simulink model "deadbeat_smm_with_lqr"  (R2015a)
settings: Solver=FixedStepDiscrete  SolverMode=SingleTasking  StartTime=0.0  StopTime=inf  FixedStep=sample_time  RelTol=1e-3
undefined symbols (not defined in the file or in its folder): A_kalman_fourbar_gear, A_kalman_transverse, A_kalman_vertical, A_lpf_accelerometer, A_lpf_fourbar_angles, A_lpf_imu, A_lpf_lateral_angle, B1_lpf_accelerometer, B1_lpf_fourbar_angles, B1_lpf_imu, B1_lpf_lateral_angle, B2_lpf_accelerometer, B2_lpf_fourbar_angles, B2_lpf_imu, B2_lpf_lateral_angle, B_dx_versus_x0, B_kalman_fourbar_gear, B_kalman_transverse, B_kalman_vertical, backwards_K_sag_of_t, backwards_P_sag_of_t, C_kalman_fourbar_gear, C_kalman_transverse, C_kalman_vertical, com_leg_motor, com_torso, contact_threshold, control_start_time, d_ankle_to_foot, d_vertical_com, desired_com_forward_velocity, desired_com_lateral_velocity, desired_initial_leg_roll_left, desired_initial_leg_roll_right, desired_stance_beta2, desired_standing_torso_pitch, desired_standing_torso_roll, desired_standing_z, desired_torso_pitch, desired_torso_roll, Discrete, enable_bouncing, fcut_contact, fdesignblkfcn, forward_dx_of_dxstar, forward_x_of_dxstar, g, gcbh, HIP_MTR_MAX_CONT_TORQUE, HIP_MTR_MAX_TORQUE, i_leg_motor, i_robot, i_torso, initial_dx_estimate, initial_dy_estimate, initial_dz_estimate, initial_leg_selection, initial_z_estimate, k_lateral_accel_for_torso_roll, k_lateral_swing_on_boom ... (+77)
libraries: simulink x21, ctrlSharedLib x7, dsparch4 x3
(part 5 of 5)

== matlab function deadbeat_smm_with_lqr/Control/Behavior Control/Primary and Lateral Behavior/Flight/Generate Parabolic Foot Trajectories ==
  data: time_remaining input; est_duration input; x_star input; y_star input; x0 input; dx0 input; y0 input; dy0 input; zdz0 input; max_parabolic_z_retraction parameter; flight input; right_left input; z_land parameter; min_f_duration parameter; X_star output size=3; Y_star output size=3; Z_star output size=3; robot_is_attached_to_boom parameter; lateral_target_position_left parameter; lateral_target_position_right parameter
%% Parabolic trajectory generation for x, y, and z
% est_duration: estimated flight time
% time_remaining: time until estimated touchdown
% stance: 1 if in stance, 0 otherwise
% x_star: desired x for foot to COM
% y_star: desired y for foot to COM
% x0: x position at takeoff
% y0: y position at takeoff
% zdz0: [z, dz] at takeoff
% max_retract: how high to lift z for ground clearance
% z_land: nominal z height for landing
% min_f_duration: minimum trajectory time

function [X_star, Y_star, Z_star]  =  ...
          GenerateParabolicFootTrajectory(time_remaining, est_duration,  ...
                               x_star, y_star, x0, dx0, y0, dy0, zdz0, ...
                               max_parabolic_z_retraction,  flight, right_left, ...
                               z_land, min_f_duration, ...
                               robot_is_attached_to_boom, lateral_target_position_left, lateral_target_position_right)

if ~flight
    X_star = [0;0;0];
    Y_star = [0;0;0];
    Z_star = [0;0;0];
    return;
end

if robot_is_attached_to_boom
    if right_left
        y_star = lateral_target_position_right;
    else
        y_star = lateral_target_position_left;
    end 
end
                           
% we are solving for yawed coordinates xyz of com-foot in flight and
% converting them to joint angles

% estimate z ballistically
% z = z_dz_liftoff(1) + z_dz_liftoff(2)*t_flight -g/2*t_flight^2;
% dz = z_dz_liftoff(2) - g*t_flight;
% 
% z = com_xdx_ydy_zdz(5); dz = com_xdx_ydy_zdz(6);
% time_remaining = (-dz-sqrt(max(dz^2 - 4*g/2*(z_land-z), 0) ) )/ (-g); % ballistic estimate of landing


  % plan a traj from init to desired in estimated duration. Use a
  % discontinuous initial condition if estimated duration too short.
  duration = max(est_duration, min_f_duration);
  t_r = max(min(time_remaining, duration),0);
  % sweep a parabola from x0 to x_star with dx_end = -dx0
  dx_star = dx0;
  x_star_t = x_star + dx_star*t_r + (x0-x_star-dx_star*duration)*(t_r/duration)^2;
  dx_star_t = -dx_star - 2*(x0-x_star-dx_star*duration)*(t_r/duration^2);
  ddx_star_t =  2*(x0-x_star-dx_star*duration)*(1/duration^2);
  
  % same for y
  dy_star = dy0;
  y_star_t = y_star + dy_star*t_r + (y0-y_star-dy_star*duration)*(t_r/duration)^2;
  dy_star_t = -dy_star - 2*(y0-y_star-dy_star*duration)*(t_r/duration^2);
  ddy_star_t =  2*(y0-y_star-dy_star*duration)*(1/duration^2);
  
  % Zero out velocities when out of time
  if time_remaining < 0
    dx_star_t = 0; ddx_star_t = 0;
    dy_star_t = 0; ddy_star_t = 0;
  end 
  
  % split duration into thirds.  First segment: parabola from z0 to
  % max_retract.  Second and third segments, cos to landing.
  z0 = zdz0(1);
  dt3 = duration / 3;
  z_min = z_land - max_parabolic_z_retraction;
  if t_r > 2*dt3;
    z_star_t = z_min + (z0-z_min)*((t_r-2*dt3)/dt3)^2;
    dz_star_t = -(z0-z_min)*2*(t_r-2*dt3)/dt3/dt3;
    ddz_star_t = (z0-z_min)*2/dt3^2;
  else
    z_star_t = z_land + (z_min-z_land)/2*(1-cos(t_r/(2*dt3)*pi));
    dz_star_t = -(z_min-z_land)/2*sin(t_r/(2*dt3)*pi)*pi/(2*dt3);
    ddz_star_t = (z_min-z_land)/2*cos(t_r/(2*dt3)*pi)*(pi/(2*dt3))^2;
  end
  
  % track a sinusoidal z of amplitude max_retract, finishing a half-cycle by t_end
  X_star = [x_star_t; dx_star_t; ddx_star_t];
  Y_star = [y_star_t; dy_star_t; ddy_star_t];
  Z_star = [z_star_t; dz_star_t; ddz_star_t];

== matlab function deadbeat_smm_with_lqr/Control/Behavior Control/Primary and Lateral Behavior/Flight/Lateral Flight Control ==
  data: hopping input; tau_primary output; tau_secondary output; RightLeftPrimary input; TorsoRoll input; LLegRoll input; RLegRoll input; Beta1_star input; Roll_star input; K_right_lat_flight parameter; K_left_lat_flight parameter; K_right_lat_flight_winch parameter; K_left_lat_flight_winch parameter; Q_phibeta1beta2 parameter; Q_phibeta1beta2_winch parameter; m_torso parameter; m_leg parameter; m_leg_motor parameter; m_total_real parameter; com_torso parameter; i_torso parameter; i_leg_motor parameter; g parameter; lateral_offset parameter; k_lateral_swing_on_boom parameter; adjusted_ref output; feedforward output; lateral_target_beta parameter; robot_is_attached_to_boom parameter
% full_state = [Roll; Beta1; Beta2; dRoll; dBeta1; dBeta2];
function [tau_primary, tau_secondary, ...
          adjusted_ref, feedforward] = lateral_flight_control(hopping, RightLeftPrimary,...
          TorsoRoll, LLegRoll, RLegRoll, Beta1_star, Roll_star,...
          K_right_lat_flight, K_left_lat_flight, K_right_lat_flight_winch, K_left_lat_flight_winch, Q_phibeta1beta2, Q_phibeta1beta2_winch,...
          m_torso, m_leg, m_leg_motor, m_total_real, com_torso, i_torso, i_leg_motor, g, lateral_offset, ...
          k_lateral_swing_on_boom, lateral_target_beta, robot_is_attached_to_boom)

    %% Define inertial quantities
    d = norm(com_torso(2:3));
    It_f = i_torso(1);
    Im_f = i_leg_motor(1); 
    phidphi = TorsoRoll; 
    symdsym = LLegRoll-RLegRoll;
    ang_mom = phidphi(2)*(m_torso*d^2 + It_f + 2*(m_leg_motor*lateral_offset^2+ Im_f)) -symdsym(2)*(m_leg_motor*lateral_offset^2+Im_f);

    %% Assign desired and measured variables 
    if RightLeftPrimary == 1
        Beta1 = RLegRoll;
        Beta2 = LLegRoll;
        Beta2_star = [lateral_target_beta; 0; 0];
    else
        Beta1 = LLegRoll;
        Beta2 = RLegRoll;
        Beta2_star = [lateral_target_beta; 0; 0];
    end    
    
    %% If robot is still on the winch, use a different set of gains
    if ~hopping
        Q_phibeta1beta2 = Q_phibeta1beta2_winch;
        K_right_lat_flight = K_right_lat_flight_winch;
        K_left_lat_flight = K_left_lat_flight_winch;
    end

    %% LQR
    ref_old = [Roll_star(1); Beta1_star(1); Beta2_star(1)];
    dref_old = [0; Beta1_star(2); Beta2_star(2)];
    ddref_old = [0; Beta1_star(3); Beta2_star(3)];
    
    % eliminate beta2 from state using momentum:
    % s_old = T*s_new+D(t); s_new = [phi; beta1];
    % dbeta_R = L/(Im_f+mm*r^2) - (It_f+mm*d^2+2*Im_f+2*mm*r^2)/(Im_f+mm*r^2)*dphi + dbeta_L 
    % beta_R = beta_R0 + L/(Im_f+mm*r^2)*t - ((It_f+mm*d^2+2*Im_f+2*mm*r^2)/(Im_f+mm*r^2)*(phi-phi0) + (beta_L-beta_L0)
    % beta_R = [beta_R0-b1*phi0-b2*beta_L0 + a*t + b1*phi + b2*beta_L;
    
    if RightLeftPrimary == 1 % beta_2 is beta_L, beta_1 is beta_R, eliminate beta2
      a = -ang_mom/(Im_f+m_leg_motor*lateral_offset^2);
      b1 = (It_f+m_torso*d^2+2*Im_f+2*m_leg_motor*lateral_offset^2)/(Im_f+m_leg_motor*lateral_offset^2); b2 = 1;
    else
      a = +ang_mom/(Im_f+m_leg_motor*lateral_offset^2);
      b1 = -(It_f+m_torso*d^2+2*Im_f+2*m_leg_motor*lateral_offset^2)/(Im_f+m_leg_motor*lateral_offset^2); b2 = 1;
    end
    
    T = [eye(2); b1, b2];
    %  D = [0; 0; 0; 0; beta_R0 - b1*phi0 - b2*beta_L0 + a*t; a];
    D = [0;0; Beta2(1) - b1*phidphi(1) - b2*Beta1(1)];
    
    % old cost (state s)  (s-s_ref)' * Q *(s-s_ref);
    % new cost (state r) =(T*r+D-s_ref)'*Q*(T*r+D-s_ref);
    %                    =(r+ (T'QT)^{-1}T'Q(D-s_ref))'*T'QT*
    %                     (r + (T'QT)^{-1}T'Q(D-s_ref))
    
    
    Q_new = T'*Q_phibeta1beta2*T;
    ref_new = Q_new\T'*Q_phibeta1beta2*(ref_old-D);
    ref_new_vel = Q_new\T'*Q_phibeta1beta2*(dref_old - [0;0; a]);
    ref_accels = Q_new\T'*Q_phibeta1beta2*(ddref_old);

    % A_phidphi_betadbeta1 = [0 1 0 0; 0 0 0 0; 0 0 0 1; 0 0 0 0];
    % assume beta1 is right
    if RightLeftPrimary == 1
        B_new_state = [0 0; 0 0; -1/(It_f+m_torso*d^2), 1/(It_f+m_torso*d^2); 1/(It_f+m_torso*d^2)+1/(Im_f+m_leg_motor*lateral_offset^2), -1/(It_f+m_torso*d^2)];
    else
        B_new_state = [0 0; 0 0; 1/(It_f+m_torso*d^2), -1/(It_f+m_torso*d^2); 1/(It_f+m_torso*d^2)+1/(Im_f+m_leg_motor*lateral_offset^2), -1/(It_f+m_torso*d^2)];
    end      
    
    %   K = lqr(A_phidphi_betadbeta1, B_phidphi_betadbeta1, Q_new, R_lat_flight);
    if RightLeftPrimary == 1
      K = K_right_lat_flight;
    else
      K = K_left_lat_flight;
    end

    new_state = [phidphi(1); Beta1(1); phidphi(2); Beta1(2)];
    new_ref_traj = [ref_new; ref_new_vel];

    feedforward = B_new_state([3 4],:)\ref_accels;
    if ~hopping, feedforward = -(m_leg_motor)*g*lateral_offset*ones(2,1); end
    tau_lqr = feedforward - K*(new_state-new_ref_traj);
    tau_1 = tau_lqr(1); tau_2 = tau_lqr(2);
    implied_beta2_star = [0 0 1]*(T*ref_new+D);
    implied_dbeta2_star = [0 0 1]*(T*ref_new_vel+[0; 0; a]);
    % implied_betadbeta2_star = [0 0 0 0 1 0; 0 0 0 0 0 1]*(T*ref_new+D);
    adjusted_ref = [ref_new; implied_beta2_star; ref_new_vel; implied_dbeta2_star];

    tau_primary = tau_1;
    tau_secondary = tau_2;
    
    
    %% When attached to boom, just do a simple PD control on lateral leg positions
    if robot_is_attached_to_boom
        tau_primary = k_lateral_swing_on_boom'*([lateral_target_beta; 0] - Beta1);
        tau_secondary = k_lateral_swing_on_boom'*([lateral_target_beta; 0] - Beta2);
    end
end

== matlab function deadbeat_smm_with_lqr/Control/Behavior Control/Primary and Lateral Behavior/Flight/Virtual Leg to Four Bar ==
  data: l_leg input; dl_leg input; ddl_leg input; phi input; dphi input; ddphi input; back output; dback output; ddback output; front output; dfront output; ddfront output
function [back, dback, ddback, front, dfront, ddfront] = VirtualLegToFourBar(l_leg, dl_leg, ddl_leg, phi, dphi, ddphi)
    [back, dback, ddback, front, dfront, ddfront] = VirtualLegToFourBar(l_leg, dl_leg, ddl_leg, phi, dphi, ddphi);
end

== matlab function deadbeat_smm_with_lqr/Control/Behavior Control/Primary and Lateral Behavior/Stance/3D Inverse Dynamics yawed ==
  data: right_or_left input; primary_leg_torque output double size=1; primary_leg_force output double size=1; torso_roll input double size=2; torso_pitch input double size=2; torso_yaw input size=2; primary_sagittal_leg_angle input size=2; primary_leg_length input size=2; primary_leg_roll input size=2; secondary_leg_roll input size=2; GRF_desired input double size=3; ddRoll_desired input double size=1; g parameter; primary_lateral_torque output double size=1; secondary_lateral_torque output double size=1; m_leg_motor parameter; m_torso parameter; i_torso parameter; i_leg_motor parameter; lateral_offset parameter; com_torso parameter; torso_centerline_roll_offset_angle parameter
%% Inverse dynamics
function [primary_leg_torque, primary_leg_force, primary_lateral_torque, secondary_lateral_torque]  =  InverseDynamics3D(right_or_left,...
                                                                                                                         torso_roll, torso_pitch, torso_yaw, ...
                                                                                                                         primary_sagittal_leg_angle, primary_leg_length, ...
                                                                                                                         primary_leg_roll, secondary_leg_roll, ...
                                                                                                                         GRF_desired, ddRoll_desired, ...
                                                                                                                         g, m_leg_motor, m_torso, i_torso, i_leg_motor, lateral_offset, com_torso, torso_centerline_roll_offset_angle)

    d = norm(com_torso(2:3));
    It = mean(i_torso);
    Im = mean(i_leg_motor);
    
    phi    = torso_roll(1) + torso_centerline_roll_offset_angle; % roll
    theta  = torso_pitch(1);                   % pitch
    alpha1 = primary_sagittal_leg_angle(1);    % primary sagittal leg angle
    beta1  = primary_leg_roll(1);              % primary leg roll
    beta2  = secondary_leg_roll(1);            % secondary leg roll
    if right_or_left
        beta1 = beta1 - torso_centerline_roll_offset_angle;
        beta2 = beta2 + torso_centerline_roll_offset_angle;
    else
        beta1 = beta1 + torso_centerline_roll_offset_angle;
        beta2 = beta2 - torso_centerline_roll_offset_angle;
    end 
    l1     = primary_leg_length(1);            % primary leg length
    
    dphi    = torso_roll(2);
    dtheta  = torso_pitch(2);
    dpsi    = torso_yaw(2);
    dalpha1 = primary_sagittal_leg_angle(2);
    dbeta1  = primary_leg_roll(2);
    dbeta2  = secondary_leg_roll(2);
    dl1     = primary_leg_length(2);

    Fx = GRF_desired(1);
    Fy = GRF_desired(2);
    Fz = GRF_desired(3);
    ddphi = ddRoll_desired;

    if right_or_left == 1
      A = A_id_roll_yawed_right(lateral_offset,d,m_leg_motor,m_torso,It,Im,phi,theta,alpha1,beta1,beta2,l1);     
      B = B_id_roll_yawed_right(lateral_offset,d,g,m_leg_motor,m_torso,It,Im,phi,theta,alpha1,beta1,beta2,l1,dphi,dtheta,dpsi,dalpha1,dbeta1,dbeta2,dl1,Fx,Fy,Fz,ddphi);
    else
      A = A_id_roll_yawed_left(lateral_offset,d,m_leg_motor,m_torso,It,Im,phi,theta,alpha1,beta1,beta2,l1);     
      B = B_id_roll_yawed_left(lateral_offset,d,g,m_leg_motor,m_torso,It,Im,phi,theta,alpha1,beta1,beta2,l1,dphi,dtheta,dpsi,dalpha1,dbeta1,dbeta2,dl1,Fx,Fy,Fz,ddphi);
    end        
    
    x_id_roll = A \ B;
    primary_leg_torque = x_id_roll(10);
    primary_lateral_torque = x_id_roll(11);
    secondary_lateral_torque = x_id_roll(12);
    primary_leg_force = x_id_roll(13);
end

== matlab function deadbeat_smm_with_lqr/Control/Behavior Control/Primary and Lateral Behavior/Stance/COM X,Y,Z  trajectory generation ==
  data: stance input; hopping input; bouncing input; x_0 output size=1; y_0 output size=1; z_ref output size=1; dz_ref output size=1; ddz_ref output size=1; x_ref output size=1; dx_ref output size=1; y_ref output size=1; dy_ref output size=1; t input size=1; dx0 input; dy0 input; target_DX input; target_DY input; z_rest_new parameter; z_amplitude parameter; spring_frequency parameter; phase_0 parameter; forward_x_of_dxstar parameter; forward_dx_of_dxstar parameter; target_dx_range parameter; T_s parameter; desired_standing_z parameter; standing_bounce_amplitude parameter; standing_bounce_w input; standing_bounce_dw input
%% COM trajectory generation for stance & foot placement for flight

% Outputs:
% x_0: desired x position for COM at touchdown
% y_0: desired y position for COM at touchdown
% [z_ref, dz_ref, ddz_ref]: reference trajectory for vertical
% [x_ref, dx_ref]: reference trajectory for forward
% [y_ref, dy_ref]: reference trajectory for lateral

% Inputs:
% t: time since touchdown
% dx0: touchdown x velocity
% dy0: touchdown y velocity
% target_DX: desired x velocity at takeoff
% s_duration: nominal stance time
% z_rest_new: z height of oscillation
% target_dx_range: full range of possible x velocities in lookup table
% forward_x_of_dxstar: master lookup table for x trajectories
% T_s: tabled vector from 0 to s_duration

function [x_0, y_0,...
          z_ref, dz_ref, ddz_ref, ...
          x_ref, dx_ref, y_ref, dy_ref] ...
          = ReferenceTrajectory(stance, hopping, bouncing, t, dx0, dy0, target_DX, target_DY, z_rest_new, z_amplitude, ...
            spring_frequency, phase_0, forward_x_of_dxstar, forward_dx_of_dxstar, ...
            target_dx_range, T_s,...
            desired_standing_z, standing_bounce_amplitude, standing_bounce_w, standing_bounce_dw)
    
    % Z trajectory 
    z_ref =  z_rest_new + z_amplitude*sin(spring_frequency*t+phase_0);
    dz_ref = z_amplitude*spring_frequency*cos(spring_frequency*t+phase_0);
    ddz_ref = -z_amplitude*spring_frequency^2*sin(spring_frequency*t+phase_0);
    
    % saturate t and initial velocity to reference library
    t_sat = max( min(t, T_s(end)), 0);

    % [X, dX] trajectory from 0 to s_duration
    forward_x_given_dxstar = squeeze(interp1(target_dx_range, forward_x_of_dxstar, target_DX));
    forward_dx_given_dxstar = squeeze(interp1(target_dx_range, forward_dx_of_dxstar, target_DX));

    dx0 = max( min(dx0, max(forward_dx_given_dxstar(:,1))), min(forward_dx_given_dxstar(:,1)) );
    x_ref  = interp2(T_s, forward_dx_given_dxstar(:,1), forward_x_given_dxstar, t_sat, dx0);
    dx_ref = interp2(T_s, forward_dx_given_dxstar(:,1), forward_dx_given_dxstar, t_sat, dx0);
    x_0 = interp1(forward_dx_given_dxstar(:,1), forward_x_given_dxstar(:,1), dx0);

    % [Y, dY] trajectory from 0 to s_duration
    % Y uses same library as X
    forward_y_given_dxstar = squeeze(interp1(target_dx_range, forward_x_of_dxstar, target_DY));
    forward_dy_given_dxstar = squeeze(interp1(target_dx_range, forward_dx_of_dxstar, target_DY));

    dy0 = max( min(dy0, max(forward_dy_given_dxstar(:,1))), min(forward_dy_given_dxstar(:,1)) );
    y_ref  = interp2(T_s, forward_dy_given_dxstar(:,1), forward_y_given_dxstar, t_sat, dy0);
    dy_ref = interp2(T_s, forward_dy_given_dxstar(:,1), forward_dy_given_dxstar, t_sat, dy0);
    y_0 = interp1(forward_dy_given_dxstar(:,1), forward_y_given_dxstar(:,1), dy0);
    
    if ~hopping && ~bouncing % Standing still
        z_ref = desired_standing_z;
        dz_ref = 0;
        ddz_ref = 0;
        x_ref = 0;
        dx_ref = 0;
        y_ref = 0;
        dy_ref =0;
    elseif ~hopping && bouncing % Bouncing while standing
        z_ref = z_rest_new + standing_bounce_amplitude*sin(t*standing_bounce_w);
        dz_ref = standing_bounce_amplitude*cos(t*standing_bounce_w)*(t*standing_bounce_dw + standing_bounce_w);
        ddz_ref = standing_bounce_amplitude*(2*standing_bounce_dw*cos(t*standing_bounce_w) - (t*standing_bounce_dw + standing_bounce_w)^2*sin(t*standing_bounce_w));
        x_ref = 0;
        dx_ref = 0;
        y_ref = 0;
        dy_ref =0;
    end
    if ~stance % Flight
        z_ref = 0;
        dz_ref = 0;
        ddz_ref = 0;
        x_ref = 0;
        dx_ref = 0;
        y_ref = 0;
        dy_ref =0;    
    end
  
end

== matlab function deadbeat_smm_with_lqr/Control/Behavior Control/Primary and Lateral Behavior/Stance/Feedback for Lateral Stabilization ==
  data: Fy_desired output; neutral_feedforward_Fy output; hopping input; stance input; right_left input; rolldroll input; symdsym input; y_dy input; beta2dbeta2 input; z_dz input; GRF_measured input; secondary_lateral_torque_desired output double size=1; m_torso parameter; m_leg_motor parameter; m_leg parameter; lateral_offset parameter; com_torso parameter; i_torso parameter; i_leg_motor parameter; desired_standing_torso_roll parameter; desired_torso_roll parameter; desired_beta2_state input; angular_momentum output; k_stance_secondary_roll parameter; k_lateral_accel_for_torso_roll parameter; g parameter; m_total_real parameter
%  x_front = [y, roll, sym, dy, droll, L]; 
function [Fy_desired,neutral_feedforward_Fy, secondary_lateral_torque_desired, angular_momentum]  =  ...
    FrontalStabilization(hopping, stance, right_left, rolldroll, symdsym, y_dy, beta2dbeta2, z_dz, GRF_measured,...
           m_torso, m_leg_motor, m_leg, lateral_offset, com_torso, i_torso, i_leg_motor, ...
           desired_standing_torso_roll, desired_torso_roll, desired_beta2_state, k_stance_secondary_roll, k_lateral_accel_for_torso_roll, g, m_total_real)
    
    % Angular momentum about the pelvis in the frontal plane
    d = norm(com_torso(2:3));
    It_f = i_torso(1);
    Im_f = i_leg_motor(1);
    lateral_robot_inertia = m_torso*d^2 + It_f + 2*(m_leg_motor*lateral_offset^2+ Im_f);
    angular_momentum = rolldroll(2)*lateral_robot_inertia - symdsym(2)*(m_leg_motor*lateral_offset^2+Im_f);
    
    % Feedforward GRFy for inverse dynamics
    neutral_feedforward_Fy = GRF_measured(3)*y_dy(1)/z_dz(1);
    
    % Desired states
    if hopping
        desired_torso_roll_state = [desired_torso_roll; 0]; 
    else
        desired_torso_roll_state = [desired_standing_torso_roll; 0];
    end
    
    % Motor torque commands
    ddz = GRF_measured(3) / m_total_real - g;
    gravity_comp = (m_leg_motor+m_leg)*lateral_offset*ddz;
    secondary_lateral_torque_desired = k_stance_secondary_roll'*(desired_beta2_state - beta2dbeta2) + gravity_comp;
    feedback_Fy = (lateral_robot_inertia * k_lateral_accel_for_torso_roll*(desired_torso_roll_state - rolldroll)) / z_dz(1);
    Fy_desired =  neutral_feedforward_Fy + feedback_Fy;
    Fy_desired = min(max(Fy_desired, -0.5*abs(GRF_measured(3))), 0.5*abs(GRF_measured(3)));
    
    if ~stance
        Fy_desired = 0;
        secondary_lateral_torque_desired = 0;
        neutral_feedforward_Fy = 0;
    end
end

== matlab function deadbeat_smm_with_lqr/Control/Behavior Control/Primary and Lateral Behavior/Stance/LQR Feedback for Desired Forward GRF ==
  data: hopping input; stance input; GRFx_desired output; netural_pitch_ff output; true_ff output; GRFx_lqr output; ddtheta_star output; ddtheta_star_neutral output; xdx input; thetadtheta input; zdz input; Fz_desired input; xdx_ref input size=2; theta_star input; K_sag input; P_sag input; measured_GRF input; Fx_disturbance input; i_robot parameter; cost_to_go output double size=1; ang_mom output; desired_standing_torso_pitch parameter; k_LQR_sagittal_infinite parameter; P_LQR_sagittal_infinite parameter
%% LQR for x state

% stance: 1 if in stance, 0 otherwise
% xdx: [ x from stance leg to COM, dx of COM]
% thetadtheta: [pitch, dpitch]
% zdz: [z of COM, dz of COM]
% Fz: Desired z GRF
% xdx_ref: [x, dx] current reference point for COM
% theta_star: desired torso pitch
% K_sag: time dependent LQR gain


% sagittal_state: [x, pitch, dx, dptich]
% theta_star: desired torso pitch


function [GRFx_desired, netural_pitch_ff, true_ff, GRFx_lqr, ddtheta_star, ddtheta_star_neutral, cost_to_go, ang_mom]  =  ...
    LQR_Sagittal(hopping, stance, xdx, thetadtheta, zdz, Fz_desired, xdx_ref, theta_star, K_sag, P_sag, measured_GRF, Fx_disturbance, i_robot,...
    desired_standing_torso_pitch, k_LQR_sagittal_infinite, P_LQR_sagittal_infinite)


    sagittal_state = [xdx(1); thetadtheta(1); xdx(2); thetadtheta(2)];
    netural_pitch_ff = measured_GRF(3)*xdx(1)/zdz(1);
    true_ff = measured_GRF(3)*xdx_ref(1)/zdz(1);
    
%     if hopping
%         sagittal_reference = [xdx_ref(1), theta_star, xdx_ref(2), 0]';
%         sagittal_error = (sagittal_state - sagittal_reference);
%         cost_to_go = 0.5*sagittal_error'*P_sag*sagittal_error;
%         GRFx_lqr = - K_sag*sagittal_error;
%         GRFx_desired = true_ff + GRFx_lqr;
%     else
        sagittal_reference = [xdx_ref(1), desired_standing_torso_pitch, xdx_ref(2), 0]';
        sagittal_error = (sagittal_state - sagittal_reference);
        cost_to_go = 0.5*sagittal_error'*P_LQR_sagittal_infinite*sagittal_error;
        %GRFx_desired = i_robot/zdz(1)*(150*(thetadtheta(1)-desired_standing_torso_pitch) + 30*thetadtheta(2)) + netural_pitch_ff;
        GRFx_lqr = - k_LQR_sagittal_infinite*sagittal_error;
        GRFx_desired = GRFx_lqr + true_ff;
%     end
    
    GRFx_desired = GRFx_desired - Fx_disturbance;
    GRFx_desired = min(max(GRFx_desired, -0.5*abs(measured_GRF(3))), 0.5*abs(measured_GRF(3))); % saturate to friction cone
    
    if stance == 0
      GRFx_lqr = 0;
      cost_to_go = 0;
      netural_pitch_ff = 0;
      true_ff = 0;
    end
    
    % quantities for logging
    ddtheta_star_neutral = -(GRFx_lqr)*zdz(1)/i_robot;
    ddtheta_star = -(GRFx_desired - netural_pitch_ff)*zdz(1)/i_robot;
    ang_mom = i_robot*thetadtheta(2);
end

== matlab function deadbeat_smm_with_lqr/Control/Behavior Control/Primary and Lateral Behavior/Stance/LQR Feedback for Desired Vertical GRF ==
  data: hopping input; stance input; zdzddz_ref input size=3; GRFz_desired output; GRFz_feedforward output; z_state input; leg_length input; Fz_disturbance input; k_LQR_vertical parameter; P_LQR_vertical parameter; m_total_real parameter; g parameter; cost_to_go output double size=1; max_leg_length parameter
%% LQR for z during stance

% stance: 1 if in stance, 0 otherwise
% z_state: [z, dz] current estimate
% zdzddz_ref: reference trajectory for z position, velocity, and acceleration


% GRFz_desired: desired z GRF
% cost_to_go: remaining LQR cost

function [GRFz_desired, GRFz_feedforward, cost_to_go]   =  ...
               LQR_Vertical_Height(hopping, stance, zdzddz_ref, z_state, leg_length, Fz_disturbance,...
                                   k_LQR_vertical, P_LQR_vertical, m_total_real, g, max_leg_length)

    z_ref = zdzddz_ref(1:2);     
    ddz_ref = zdzddz_ref(3);
    z_error = (z_state - z_ref);
    GRFz_feedforward = m_total_real*(g+ddz_ref);
    GRFz_desired = GRFz_feedforward - k_LQR_vertical*z_error;
    GRFz_desired = GRFz_desired - Fz_disturbance;
    GRFz_desired = max(0, GRFz_desired); % No negative vertical GRFs
    
    if hopping
        if z_ref(2) < 0
            GRFz_desired = max(50, GRFz_desired); % prevent foot from slipping
        elseif leg_length(1) >= max_leg_length
            GRFz_desired = 0; % prevent hyperextension
        end
    else % standing bounce
        GRFz_desired = max(100, GRFz_desired); % prevent lift off
    end
    
    cost_to_go = z_error'*P_LQR_vertical*z_error;
    
    if stance == 0
      GRFz_desired = 0;
      cost_to_go = 0;
    end
end

== matlab function deadbeat_smm_with_lqr/Control/Behavior Control/Primary and Lateral Behavior/Stance/Limit Lateral Knee Torque ==
  data: Fy_s input; Fy_command output; Fz_s input; y_knee_front input; Fz_command output; y_knee_back input; z_knee_front input; z_knee_back input; max_lateral_knee_torque parameter
% Optimally limit lateral torque about the knee joint
function [Fy_command, Fz_command] = limit_knee_torque(Fy_s, Fz_s, y_knee_front, y_knee_back, z_knee_front, z_knee_back, max_lateral_knee_torque)

    s = max_lateral_knee_torque;
    zf = z_knee_front;
    yf = y_knee_front;
    zb = z_knee_back;
    yb = y_knee_back;
    front_knee_torque = abs(yf*Fz_s - zf*Fy_s);
    back_knee_torque = abs(yb*Fz_s - zb*Fy_s);
    y = yf;
    z = zf;
    if front_knee_torque < back_knee_torque
        y = yb;
        z = zb;
    end
    lambda1 = 10;
    lambda2 = 1;

    % possible solutions
    Fz = [  (lambda2*s*y + Fz_s*lambda1*z^2 + Fy_s*lambda2*y*z)/(lambda2*y^2 + lambda1*z^2);
            (Fz_s*lambda1*z^2 - lambda2*s*y + Fy_s*lambda2*y*z)/(lambda2*y^2 + lambda1*z^2);
            Fz_s];

    Fy = [  (Fy_s*lambda2*y^2 - lambda1*s*z + Fz_s*lambda1*y*z)/(lambda2*y^2 + lambda1*z^2);
            (lambda1*s*z + Fy_s*lambda2*y^2 + Fz_s*lambda1*y*z)/(lambda2*y^2 + lambda1*z^2);
            Fy_s];

    % test constraints (with some margin for numerical error)
    c1 = s - y*Fz + z*Fy >= -1;
    c2 = s + y*Fz - z*Fy >= -1;
    constraints = c1 & c2;

    % maximize objective function
    f = -lambda1*(Fz_s - Fz).^2-lambda2*(Fy_s - Fy).^2;
    satisfied = find(constraints);
    if size(f(satisfied),1) == 0
      satisfied = [1; 2];
    end
    [~,I] = max(f(satisfied));
    Fz_command = Fz(satisfied(I));
    Fy_command = Fy(satisfied(I));
end

== matlab function deadbeat_smm_with_lqr/Control/Behavior Control/Primary and Lateral Behavior/Stance/Lookup finite horizon LQR gain ==
  data: K_sag output size=[1,4]; P_sag output size=[4,4]; t_forward input; backwards_K_sag_of_t parameter; T_lqr parameter; stance_duration parameter; backwards_P_sag_of_t parameter
%% Interpolates pregenerated finite horizon LQR gain tables 
% sagittal_state: [X, Pitch, dX, dPtich]
% frontal state: [Y; Roll; sym; dY; dRoll; angular_momentum];
function [K_sag, P_sag]  =  FiniteHorizonLQRLookup(t_forward, backwards_K_sag_of_t, T_lqr, stance_duration, backwards_P_sag_of_t)
  t = stance_duration - t_forward; % gains are scheduled w.r.t time until end.                                     
  t = min(max(t, min(T_lqr)), max(T_lqr));
  K_sag = interp1(T_lqr, backwards_K_sag_of_t, t);
  P_sag = squeeze(interp1(T_lqr,backwards_P_sag_of_t,t));
end

== matlab function deadbeat_smm_with_lqr/Control/Behavior Control/Primary and Lateral Behavior/Stance/Torque Distribution/Motor Torque Saturation Optimization ==
  data: x1s input; t1 output; x2s input; lambda1 parameter; lambda2 parameter; max_torque_sagittal parameter; t2 output
% Optimal leg motor torque distribution
function [t1, t2] = distribute_torque(x1s, x2s, lambda1, lambda2, max_torque_sagittal)

s = max_torque_sagittal;

% possible solutions
x1 = [                                                      x1s;
                                                            0;
                                                            s;
                                                            0;
                                                           -s;
  (lambda2*s + lambda1*x1s - lambda2*x2s)/(lambda1 + lambda2);
  (lambda1*x1s - lambda2*s + lambda2*x2s)/(lambda1 + lambda2);
  (lambda2*s + lambda1*x1s + lambda2*x2s)/(lambda1 + lambda2);
 -(lambda2*s - lambda1*x1s + lambda2*x2s)/(lambda1 + lambda2)];
 
x2 = [                                                      x2s;
                                                            s;
                                                            0;
                                                           -s;
                                                            0;
  (lambda1*s - lambda1*x1s + lambda2*x2s)/(lambda1 + lambda2);
  (lambda1*s + lambda1*x1s + lambda2*x2s)/(lambda1 + lambda2);
  (lambda1*x1s - lambda1*s + lambda2*x2s)/(lambda1 + lambda2);
 -(lambda1*s + lambda1*x1s - lambda2*x2s)/(lambda1 + lambda2)];

% test constraints
c1 = s - x1 - x2 >= 0;
c2 = s + x1 + x2 >= 0;
c3 = s - x1 + x2 >= 0;
c4 = s + x1 - x2 >= 0;
constraints = c1 & c2 & c3 & c4;

% objective function to maximize
f = -lambda1*(x1-x1s).^2-lambda2*(x2-x2s).^2;
satisfied = find(constraints);
[~,I] = max(f(satisfied));

t1 = x1(satisfied(I));
t2 = x2(satisfied(I));

== matlab function deadbeat_smm_with_lqr/Control/Behavior Control/Primary and Lateral Behavior/Stance/X & Pitch State Disturbance Observer Error-Proportional ==
  data: enabled input; Fx input size=1; z_dz input; d_hat_tp1 output size=1; x_dx input size=2; theta_dtheta input; sample_time parameter; m_total_real parameter; g parameter; i_robot parameter
function d_hat_tp1 = disturbance_observer(enabled, Fx, z_dz, x_dx, theta_dtheta, sample_time, m_total_real, g, i_robot)
    
    order = 2;
    L = 2*2.^[1:order+1] .* factorial(order+1)./(factorial(order+1-(1:(order+1))).*factorial(1:order+1));

    persistent z_t d_hat_t integral_term;
    if isempty(z_t) || enabled
        z_t = 0;
        d_hat_t = 0;
        integral_term = zeros(order,1);
    end
    
%     persistent z_t;
%     if isempty(z_t) || enabled
%         z_t = 0;
%     end

    % Define system
    A_d = [ 1, 0, sample_time, 0;
            0, 1, 0, sample_time;
            0, 0, 1, 0;
            m_total_real*g*sample_time/i_robot, 0, 0, 1];
    Bu_d = [0; 0; sample_time/m_total_real; -sample_time*z_dz(1)/i_robot];
    A_c = [ 0, 0, 1, 0;
            0, 0, 0, 1;
            0, 0, 0, 0;
            m_total_real*g/i_robot, 0, 0, 0];
    Bu_c = [0; 0; 1/m_total_real; -z_dz(1)/i_robot];
    Bd_c = [0; 0; 1/m_total_real; -z_dz(1)/i_robot];
    %L = L_dob_xdx_thetadtheta;
    x = [x_dx(1); theta_dtheta(1); x_dx(2); theta_dtheta(2)];
    u = Fx;

%     % Estimate disturbance
%     x_tp1 = A_d*x + Bu_d*u;
%     z_tp1 = z_t - sample_time*L*(Bd_c*(z_t + L*x) + A_c*x + Bu_c*u);
%     d_hat_tp1 = z_tp1 + L*x_tp1;
%     z_t = z_tp1;

    % Estimate disturbance
    z_tp1 = z_t + sample_time*(pinv(Bd_c)*(A_c*x + Bu_c*u) + d_hat_t);
    x_tp1 = A_d*x + Bu_d*u;
    integral_term(1) = integral_term(1) + sample_time*(pinv(Bd_c)*x_tp1 - z_tp1);
    for i=2:order
        integral_term(i) = integral_term(i) + sample_time*integral_term(i-1);
    end
    d_hat_tp1 = L*[(pinv(Bd_c)*x_tp1 - z_tp1); integral_term];
    d_hat_t = d_hat_tp1;
    z_t = z_tp1;
    
    
end

== matlab function deadbeat_smm_with_lqr/Control/Behavior Control/Primary and Lateral Behavior/Stance/Z State Disturbance Observer Error-Proportional ==
  data: enabled input; Fz input size=1; d_hat_tp1 output size=1; z_dz input size=2; m_total_real parameter; g parameter; sample_time parameter
function d_hat_tp1  = disturbance_observer(enabled, Fz, z_dz, m_total_real, g, sample_time)

    order = 2;
    L = 2*2.^[1:order+1] .* factorial(order+1)./(factorial(order+1-(1:(order+1))).*factorial(1:order+1));

    persistent z_t d_hat_t integral_term;
    if isempty(z_t) || enabled
        z_t = 0;
        d_hat_t = 0;
        integral_term = zeros(order,1);
    end
   
    % Define system
    A_d = [1, sample_time; 0, 1];
    Bu_d = [0; sample_time/m_total_real];
    A_c = [0 1; 0 0];
    Bu_c = [0; 1/m_total_real];
    Bd_c = [0; 1/m_total_real];
    x = z_dz;
    u = Fz - m_total_real*g;
 
    % Estimate disturbance
    z_tp1 = z_t + sample_time*(pinv(Bd_c)*(A_c*x + Bu_c*u) + d_hat_t);
    x_tp1 = A_d*x + Bu_d*u;
    integral_term(1) = integral_term(1) + sample_time*(pinv(Bd_c)*x_tp1 - z_tp1);
    for i=2:order
        integral_term(i) = integral_term(i) + sample_time*integral_term(i-1);
    end
    d_hat_tp1 = L*[(pinv(Bd_c)*x_tp1 - z_tp1); integral_term];
    d_hat_t = d_hat_tp1;
    z_t = z_tp1;
    
end

== matlab function deadbeat_smm_with_lqr/Control/Behavior Control/Primary and Lateral Behavior/ToggleRightLeftLeg ==
  data: toggle input boolean; direction output double; previous input double
function direction = TogglePositiveNegative(toggle, previous)
    
    if toggle
        direction = -previous;
    else
        direction = previous;
    end

end

== matlab function deadbeat_smm_with_lqr/Control/Compute Body Frame Accelerations/Convert to Body Frame IMU Accelerations ==
  data: accelerometer input; imu_accelerations output; g parameter
function imu_accelerations = imu_to_body_frame(accelerometer, g)
    z_up_rotation = [1, 0, 0; 0, 0, 1; 0, -1, 0];
    align_xy_rotation = [sqrt(2)/2, -sqrt(2)/2, 0; sqrt(2)/2, sqrt(2)/2, 0; 0, 0, 1];
    imu_accelerations = g*z_up_rotation*align_xy_rotation*accelerometer;
end

== matlab function deadbeat_smm_with_lqr/Control/Behavior Control/Compute COM Translational Acceleration (IMU uses non-rotating measurement frame) ==
  data: com_acceleration_world output; torso_angular_accelerations input; imu_translational_accelerations_body input; torso_roll input; torso_pitch input; torso_yaw input; com_position_world input; com_velocity_world input; hip_roll_accelerations input; right_hip_roll input; left_hip_roll input; pelvis_to_imu parameter; com_torso parameter; com_leg_motor parameter; m_leg_motor parameter; m_leg parameter; m_torso parameter; torso_com_acceleration_world output; pelvis_acceleration_world output; right_hip_acceleration_world output; left_hip_acceleration_world output; com_acceleration_yawed output; g parameter
function [com_acceleration_world, torso_com_acceleration_world, pelvis_acceleration_world, right_hip_acceleration_world, left_hip_acceleration_world, com_acceleration_yawed] ...
          = compute_com_acceleration(torso_angular_accelerations, imu_translational_accelerations_body, torso_roll, torso_pitch, torso_yaw, ...
          com_position_world, com_velocity_world, ...
          hip_roll_accelerations, right_hip_roll, left_hip_roll, pelvis_to_imu, com_torso, com_leg_motor, m_leg_motor, m_leg, m_torso, g)

    % Body frame to Yawed frame rotations  
    R_body_to_yawed = R_pitch(torso_pitch(1))*R_roll(torso_roll(1));
    dR_body_to_yawed = dR_pitch(torso_pitch(1),torso_pitch(2))*R_roll(torso_roll(1)) + R_pitch(torso_pitch(1))*dR_roll(torso_roll(1),torso_roll(2));
    ddR_body_to_yawed = ddR_pitch(torso_pitch(1),torso_pitch(2),torso_angular_accelerations(2))*R_roll(torso_roll(1)) ...
                        + R_pitch(torso_pitch(1))*ddR_roll(torso_roll(1),torso_roll(2),torso_angular_accelerations(1)) ... 
                        + 2*dR_pitch(torso_pitch(1),torso_pitch(2))*dR_roll(torso_roll(1),torso_roll(2));
    % Yawed frame to World frame rotations  
    R_yawed_to_world = R_yaw(torso_yaw(1));
    dR_yawed_to_world = dR_yaw(torso_yaw(1),torso_yaw(2));
    ddR_yawed_to_world = ddR_yaw(torso_yaw(1),torso_yaw(2),torso_angular_accelerations(3));
    % Compute translational acceleration of torso COM
    R_position_body_to_world = R_yawed_to_world*R_body_to_yawed;
    R_velocity_body_to_world = dR_yawed_to_world*R_body_to_yawed + R_yawed_to_world*dR_body_to_yawed;
    R_acceleration_body_to_world = ddR_yawed_to_world*R_body_to_yawed + 2*dR_yawed_to_world*dR_body_to_yawed + R_yawed_to_world*ddR_body_to_yawed;
    imu_to_torso_com_acceleration_world = R_acceleration_body_to_world*(com_torso - pelvis_to_imu)';
    imu_acceleration_world = R_yawed_to_world*R_body_to_yawed*imu_translational_accelerations_body;
    torso_com_acceleration_world = imu_acceleration_world + imu_to_torso_com_acceleration_world;
    % Compute accelerations of hip COMs
    R_right_hip_to_body =     R_roll(-pi/2+right_hip_roll(1));
    dR_right_hip_to_body =   dR_roll(-pi/2+right_hip_roll(1), right_hip_roll(2));
    ddR_right_hip_to_body = ddR_roll(-pi/2+right_hip_roll(1), right_hip_roll(2), hip_roll_accelerations(1));
    R_left_hip_to_body =     R_roll(pi/2-left_hip_roll(1));
    dR_left_hip_to_body =   dR_roll(pi/2-left_hip_roll(1), -left_hip_roll(2));
    ddR_left_hip_to_body = ddR_roll(pi/2-left_hip_roll(1), -left_hip_roll(2), -hip_roll_accelerations(2));
    imu_to_pelvis_com_acceleration_world = R_acceleration_body_to_world*(-pelvis_to_imu)';  
    pelvis_acceleration_world = imu_acceleration_world + imu_to_pelvis_com_acceleration_world;
    left_hip_acceleration_world = pelvis_acceleration_world + (R_acceleration_body_to_world*R_left_hip_to_body + 2*R_velocity_body_to_world*dR_left_hip_to_body + R_position_body_to_world*ddR_left_hip_to_body)*com_leg_motor';
    right_hip_acceleration_world = pelvis_acceleration_world + (R_acceleration_body_to_world*R_right_hip_to_body + 2*R_velocity_body_to_world*dR_right_hip_to_body + R_position_body_to_world*ddR_right_hip_to_body)*(com_leg_motor.*[1,-1,1])';
    % Compute total system COM acceleration
    m_hip = m_leg+m_leg_motor;
    m_total = 2*m_hip + m_torso;
    com_acceleration_world = (m_torso*torso_com_acceleration_world + m_hip*(left_hip_acceleration_world + right_hip_acceleration_world))/m_total;
    com_acceleration_yawed = ddR_yawed_to_world'*com_position_world + 2*dR_yawed_to_world'*com_velocity_world + R_yawed_to_world'*com_acceleration_world;
    com_acceleration_yawed(3) = com_acceleration_yawed(3) - g;
end

function R_yp = R_pitch(theta) % map from pitched to yawed
  R_yp = [cos(theta), 0, sin(theta); ...
          0, 1, 0; ...
          -sin(theta), 0, cos(theta)];
end
function dR_yp = dR_pitch(theta,dtheta)
  dR_yp = dtheta*[-sin(theta), 0, cos(theta); ...
                  0, 0, 0; ... 
                  -cos(theta), 0, -sin(theta)];
end
function ddR_yp = ddR_pitch(theta,dtheta,ddtheta)
  ddR_yp = ddtheta*[-sin(theta), 0, cos(theta); ...
                    0, 0, 0; ... 
                    -cos(theta), 0, -sin(theta)] ...
           + dtheta^2*[-cos(theta), 0, -sin(theta); ...
                     0, 0, 0; ...
                     sin(theta), 0, -cos(theta)];
end
function R_pr = R_roll(phi) % map from rolled to pitched
  R_pr = [1, 0, 0; ...
          0, cos(phi), -sin(phi); ...
          0, sin(phi), cos(phi)]; 
end
function dR_pr = dR_roll(phi,dphi)
  dR_pr = dphi*[0, 0, 0; ...
                0, -sin(phi), -cos(phi); ...
                0, cos(phi), -sin(phi)];
end
function ddR_pr = ddR_roll(phi, dphi, ddphi)
  ddR_pr = ddphi*[0, 0, 0; ...
                  0, -sin(phi), -cos(phi); ...
                  0, cos(phi), -sin(phi)] ...
           + dphi^2*[0, 0, 0; ...
                   0, -cos(phi), sin(phi);...
                   0, -sin(phi), -cos(phi)];
end
function R_gy = R_yaw(psi) % map yawed frame to global
  R_gy = [cos(psi), -sin(psi), 0; sin(psi), cos(psi), 0; 0 0 1]; 
end
function dR_gy = dR_yaw(psi,dpsi)
  dR_gy = dpsi*[-sin(psi), -cos(psi), 0; cos(psi), -sin(psi), 0; 0 0 0];
end
function ddR_gy = ddR_yaw(psi,dpsi,ddpsi)
  ddR_gy = ddpsi*[-sin(psi), -cos(psi), 0; cos(psi), -sin(psi), 0; 0 0 0] ...
           + dpsi^2*[-cos(psi), sin(psi), 0; -sin(psi), -cos(psi), 0; 0 0 0];
end

== matlab function deadbeat_smm_with_lqr/Control/Behavior Control/State Estimation/ComputeKneePositions ==
  data: roll input; pitch input; yaw input; left_leg_sagittal_angle input; left_leg_lateral_angle input; left_leg_length input; right_leg_sagittal_angle input; right_leg_lateral_angle input; right_leg_length input; right_back_angle input; left_back_angle input; right_front_angle input; left_front_angle input; m_torso parameter; m_leg_motor parameter; m_leg parameter; com_torso parameter; com_leg_motor parameter; lateral_offset parameter; front_knee_to_right_foot output; back_knee_to_right_foot output; front_knee_to_left_foot output; back_knee_to_left_foot output
function [front_knee_to_right_foot, back_knee_to_right_foot,...
          front_knee_to_left_foot, back_knee_to_left_foot] = ...
         KneePositionsUsingKinematics(roll, pitch, yaw, ...
                                    left_leg_sagittal_angle, left_leg_lateral_angle, left_leg_length, ...
                                    right_leg_sagittal_angle, right_leg_lateral_angle, right_leg_length, ...
                                    right_back_angle, left_back_angle, right_front_angle, left_front_angle,...
                                    m_torso, m_leg_motor, m_leg, com_torso, com_leg_motor, lateral_offset)
                    
    q =  [roll(1), pitch(1), yaw(1), left_leg_sagittal_angle(1), left_leg_lateral_angle(1), left_leg_length(1), right_leg_sagittal_angle(1), right_leg_lateral_angle(1), right_leg_length(1)];
    dq = [roll(2), pitch(2), yaw(2), left_leg_sagittal_angle(2), left_leg_lateral_angle(2), left_leg_length(2), right_leg_sagittal_angle(2), right_leg_lateral_angle(2), right_leg_length(2)];                
    [ ~, ~, left_foot_to_com, ~, right_foot_to_com, ~ ] = ComCalculationFromRobot( q, dq, m_torso, m_leg_motor, m_leg, com_torso, com_leg_motor, lateral_offset );

    q =  [roll(1), pitch(1), yaw(1), left_front_angle(1), left_leg_lateral_angle(1), 0.5, right_front_angle(1), right_leg_lateral_angle(1), 0.5];
    dq = [roll(2), pitch(2), yaw(2), left_front_angle(2), left_leg_lateral_angle(2), 0, right_front_angle(2), right_leg_lateral_angle(2), 0];   
    [ ~, ~, left_front_knee_to_com, ~, right_front_knee_to_com, ~ ] = ComCalculationFromRobot( q, dq, m_torso, m_leg_motor, m_leg, com_torso, com_leg_motor, lateral_offset );
    
    q =  [roll(1), pitch(1), yaw(1), left_back_angle(1), left_leg_lateral_angle(1), 0.4, right_back_angle(1), right_leg_lateral_angle(1), 0.4];
    dq = [roll(2), pitch(2), yaw(2), left_back_angle(2), left_leg_lateral_angle(2), 0, right_back_angle(2), right_leg_lateral_angle(2), 0];   
    [ ~, ~, left_back_knee_to_com, ~, right_back_knee_to_com, ~ ] = ComCalculationFromRobot( q, dq, m_torso, m_leg_motor, m_leg, com_torso, com_leg_motor, lateral_offset );
   
    front_knee_to_left_foot = left_front_knee_to_com(4:6) - left_foot_to_com(4:6);
    front_knee_to_right_foot = right_front_knee_to_com(4:6) - right_foot_to_com(4:6);
    back_knee_to_left_foot = left_back_knee_to_com(4:6) - left_foot_to_com(4:6);
    back_knee_to_right_foot = right_back_knee_to_com(4:6) - right_foot_to_com(4:6);
end

== matlab function deadbeat_smm_with_lqr/Control/Behavior Control/State Estimation/Kalman Filtering/Measurement Noise Covariance Matricies ==
  data: R_transverse output; vertical_GRF_L input; vertical_GRF_R input; R_kalman_foot_stance parameter; R_kalman_foot_slip parameter; R_kalman_accelerometer parameter; sample_time parameter; m_total_real parameter; g parameter; R_vertical output; kalman_stance_slip_threshold parameter
function [R_transverse, R_vertical] =...
         MeasurementNoiseCovariance(vertical_GRF_L, vertical_GRF_R, ...
           R_kalman_foot_stance, R_kalman_foot_slip, R_kalman_accelerometer, sample_time, m_total_real, g, kalman_stance_slip_threshold)

    % filter states: [dx_w]; [dy_w]; [dz_w];
    % measurements:  [dx_w-dfL + dfL_hat; dx_w-dfR + dfR_hat]; 

    ratio_L = max(0, min(vertical_GRF_L/(kalman_stance_slip_threshold*m_total_real*g),1)); % ratio is 0 if no load, 1 if at least equilibrium
    ratio_R = max(0, min(vertical_GRF_R/(kalman_stance_slip_threshold*m_total_real*g),1));
    R_transverse = diag([ratio_L*R_kalman_foot_stance + (1-ratio_L)*R_kalman_foot_slip, ...
                         ratio_R*R_kalman_foot_stance + (1-ratio_R)*R_kalman_foot_slip, ...
                         R_kalman_accelerometer])/sample_time;
    R_vertical = diag([ratio_L*R_kalman_foot_stance  + (1-ratio_L)*R_kalman_foot_slip,...
                       ratio_R*R_kalman_foot_stance  + (1-ratio_R)*R_kalman_foot_slip,...
                       R_kalman_accelerometer])/sample_time;
end

== matlab function deadbeat_smm_with_lqr/Control/Behavior Control/State Estimation/Kalman Filtering/eigen values ==
  data: Z input; E output
function E = eigen(Z)
    E = real(eig(Z));
    E = sort(E);
end

== matlab function deadbeat_smm_with_lqr/Control/Behavior Control/State Estimation/Kalman Filtering/eigen values1 ==
  data: Z input; E output
function E = eigen(Z)
    E = real(eig(Z));
    E = sort(E);
end

== matlab function deadbeat_smm_with_lqr/Control/Behavior Control/State Estimation/Kalman Filtering/eigen values2 ==
  data: Z input; E output
function E = eigen(Z)
    E = real(eig(Z));
    E = sort(E);
end

== matlab function deadbeat_smm_with_lqr/Control/Behavior Control/State Estimation/PositionUsingRobotGeometry ==
  data: com_left_foot output; dcom_left_foot output; com_right_foot output; dcom_right_foot output; right_left input; horizontal_com_position output; roll input; pitch input; yaw input; horizontal_com_velocity output; lateral_com_position output; lateral_com_velocity output; left_leg_sagittal_angle input; left_leg_lateral_angle input; left_leg_length input; right_leg_sagittal_angle input; right_leg_lateral_angle input; right_leg_length input; m_torso parameter; m_leg_motor parameter; m_leg parameter; com_torso parameter; com_leg_motor parameter; lateral_offset parameter; vertical_com_position output; vertical_com_velocity output; com_pelvis output; dcom_pelvis output
% Returns 2D COM relative to primary foot
function [com_left_foot, dcom_left_foot, com_right_foot, dcom_right_foot,...
          horizontal_com_position, horizontal_com_velocity, ...
          lateral_com_position, lateral_com_velocity, ...
          vertical_com_position, vertical_com_velocity, ...
          com_pelvis, dcom_pelvis] = ...
         ComPositionUsingRobotGeometry(right_left, ...
                                    roll, pitch, yaw, ...
                                    left_leg_sagittal_angle, left_leg_lateral_angle, left_leg_length, ...
                                    right_leg_sagittal_angle, right_leg_lateral_angle, right_leg_length, ...
                                    m_torso, m_leg_motor, m_leg, com_torso, com_leg_motor, lateral_offset)
                    
    q =  [roll(1), pitch(1), yaw(1), left_leg_sagittal_angle(1), left_leg_lateral_angle(1), left_leg_length(1), right_leg_sagittal_angle(1), right_leg_lateral_angle(1), right_leg_length(1)];
    dq = [roll(2), pitch(2), yaw(2), left_leg_sagittal_angle(2), left_leg_lateral_angle(2), left_leg_length(2), right_leg_sagittal_angle(2), right_leg_lateral_angle(2), right_leg_length(2)];
                    
    [ com_pelvis, dcom_pelvis, ...
      com_left_foot, dcom_left_foot, ...
      com_right_foot, dcom_right_foot ] = ...
    ComCalculationFromRobot( q, dq, m_torso, m_leg_motor, m_leg, com_torso, com_leg_motor, lateral_offset );

    if right_left
        com_position = com_right_foot(4:6);
        com_velocity = dcom_right_foot(4:6);
    else
        com_position = com_left_foot(4:6);
        com_velocity = dcom_left_foot(4:6);
    end


    horizontal_com_position = com_position(1);
    horizontal_com_velocity = com_velocity(1);
    lateral_com_position = com_position(2);
    lateral_com_velocity = com_velocity(2);
    vertical_com_position = com_position(3);
    vertical_com_velocity = com_velocity(3);

end
